simulink model "OneZone_STD2004_Buffalo_TypOcc"  (R2020a)
settings: Solver=FixedStepAuto  StartTime=15638400  StopTime=15811200  FixedStep=60  RelTol=1e-3
settings Model: Creator=zhelu  LastModifiedBy=yl3328

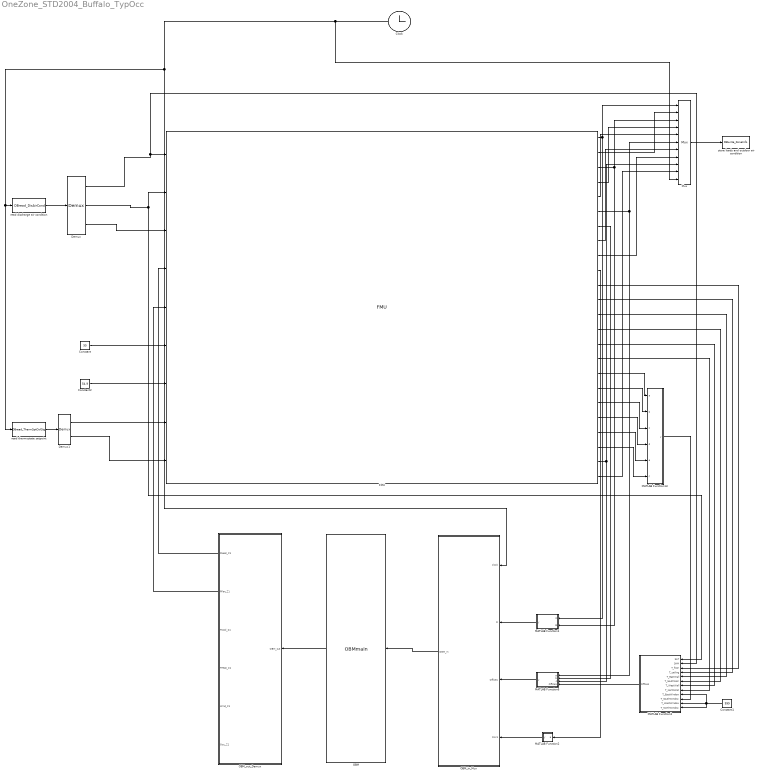
== system OneZone_STD2004_Buffalo_TypOcc ==
  Clock : Clock
  Constant : Constant  Value=55
  Constant1 : Constant  Value=999
  Constant2 : Constant  Value=54.9
  Demux : Demux  Outputs=3
  Demux1 : Demux  Outputs=2
  FMU : FMU  FMUName=ASHRAE901_OfficeSmall_STD2004_Buffalo.fmu  FMUMode=CoSimulation
      mask Type: ASHRAE901_OfficeSmall_STD2004_Buffalo.idf [Co-Simulation, v2.0]
      mask Display:
      | disp('ASHRAE901_OfficeSmall_STD2004_Buffalo.idf');
      | port_label('output',1,'T_out');
      | port_label('output',2,'DewpointT_out');
      | port_label('output',3,'RH_out');
      | port_label('output',4,'Perimeter_ZN_1_SenLoads');
      | port_label('output',5,'Perimeter_ZN_1_LatLoads');
      | port_label('output',6,'Perimeter_ZN_1_Temp');
      | port_label('output',7,'Perimeter_ZN_1_RadTemp');
      | port_label('output',8,'Perimeter_ZN_1_DewpointT');
      | port_label('output',9,'Perimeter_ZN_1_HumdRat');
      | port_label('output',10,'Perimeter_ZN_1_Occ');
      | port_label('output',11,'Perimeter_ZN_1_FLOOR_T');
      | port_label('output',12,'Perimeter_ZN_1_CEILING_T');
      | port_label('output',13,'Perimeter_ZN_1_WALL_EAST_T');
      | port_label('output',14,'Perimeter_ZN_1_WALL_SOUTH_T');
      | port_label('output',15,'Perimeter_ZN_1_WALL_WEST_T');
      | port_label('output',16,'Perimeter_ZN_1_WALL_NORTH_T');
      | port_label('output',17,'Perimeter_ZN_1_WALL_SOUTH_WINDOW1_T');
      | port_label('output',18,'Perimeter_ZN_1_WALL_SOUTH_WINDOW2_T');
      | port_label('output',19,'Perimeter_ZN_1_WALL_SOUTH_WINDOW3_T');
      | port_label('output',20,'Perimeter_ZN_1_WALL_SOUTH_WINDOW4_T');
      | port_label('output',21,'Perimeter_ZN_1_WALL_SOUTH_WINDOW5_T');
      | port_label('output',22,'Perimeter_ZN_1_WALL_SOUTH_WINDOW6_T');
      | port_label('output',23,'Perimeter_ZN_1_RelaHumd');
      | port_label('output',24,'w_out');
      | port_label('input',1,'Perimeter_ZN_1 SupplyFlow');
      | port_label('input',2,'Perimeter_ZN_1 SupplyTemp');
      | port_label('input',3,'Perimeter_ZN_1 SupplyHumd');
      | port_label('input',4,'Perimeter_ZN_1_PHeat');
      | port_label('input',5,'Perimeter_ZN_1_PFan');
      | port_label('input',6,'Perimeter_ZN_1_TCool');
      | port_label('input',7,'Perimeter_ZN_1_THeat');
      | port_label('input',8,'OtherZN_TC');
      | port_label('input',9,'OtherZN_TH');
  MATLAB Function1 : MATLAB Function  TreatAsAtomicUnit=on
  MATLAB Function13 : MATLAB Function  TreatAsAtomicUnit=on
  MATLAB Function2 : MATLAB Function  TreatAsAtomicUnit=on
  MATLAB Function3 : MATLAB Function  TreatAsAtomicUnit=on
  MATLAB Function6 : MATLAB Function  TreatAsAtomicUnit=on
  Mux : Mux  Inputs=11
  OBM : M-S-Function  FunctionName=OBMmain
  OBM_in_Mux : MATLAB Function  TreatAsAtomicUnit=on
  OBM_out_Demux : MATLAB Function  TreatAsAtomicUnit=on
  read discharge air condition : M-S-Function  FunctionName=DBread_DisAirCond
  read thermostate setpoint : M-S-Function  FunctionName=DBread_ThermSptCtrlSig
  store loads and outdoor air condition : M-S-Function  FunctionName=DBwrite_ZoneInfo
  wires:
  Mux/1 -> store loads and outdoor air condition/1
  read discharge air condition/1 -> Demux/1
  Clock/1 -> Mux/11, read thermostate setpoint/1, read discharge air condition/1, OBM_in_Mux/1(clock)
  MATLAB Function1/1(y) -> OBM_in_Mux/2(O)
  MATLAB Function6/1(y) -> OBM_in_Mux/3(Office1)
  MATLAB Function2/1(y) -> OBM_in_Mux/4(Occ1)
  OBM_in_Mux/1(OBM_in) -> OBM/1
  OBM/1 -> OBM_out_Demux/1(OBM_out)
  OBM_out_Demux/1(PHeat_Z1) -> FMU/4
  OBM_out_Demux/2(PFan_Z1) -> FMU/5
  Constant2/1 -> FMU/7
  Constant/1 -> FMU/6
  Demux/1 -> MATLAB Function3/2(SAM), FMU/1
  Demux/2 -> MATLAB Function3/1(SAT), FMU/2
  Demux/3 -> FMU/3
  FMU/1 -> Mux/1, MATLAB Function1/1(A)
  FMU/3 -> MATLAB Function1/2(B), Mux/3
  FMU/10 -> MATLAB Function2/1(a)
  FMU/6 -> MATLAB Function6/1(a), Mux/6
  FMU/7 -> MATLAB Function6/2(b)
  FMU/9 -> Mux/8
  FMU/2 -> Mux/2
  FMU/4 -> Mux/4
  FMU/5 -> Mux/5
  FMU/8 -> Mux/7
  FMU/11 -> MATLAB Function3/3(T_floor)
  FMU/12 -> MATLAB Function3/4(T_ceiling)
  FMU/13 -> MATLAB Function3/5(T_EastWall)
  FMU/14 -> MATLAB Function3/6(T_SouthWall)
  FMU/15 -> MATLAB Function3/7(T_WestWall)
  FMU/16 -> MATLAB Function3/8(T_NorthWall)
  FMU/17 -> MATLAB Function13/1(a)
  FMU/18 -> MATLAB Function13/2(b)
  FMU/19 -> MATLAB Function13/3(c)
  FMU/20 -> MATLAB Function13/4(d)
  FMU/21 -> MATLAB Function13/5(e)
  FMU/22 -> MATLAB Function13/6(f)
  MATLAB Function13/1(y) -> MATLAB Function3/10(T_SouthWindow)
  Constant1/1 -> MATLAB Function3/12(T_NorthWindow), MATLAB Function3/9(T_EastWindow), MATLAB Function3/11(T_WestWindow)
  MATLAB Function3/1(Office1) -> MATLAB Function6/4(Office1)
  FMU/23 -> MATLAB Function6/3(c), Mux/9
  FMU/24 -> Mux/10
  read thermostate setpoint/1 -> Demux1/1
  Demux1/1 -> FMU/8
  Demux1/2 -> FMU/9

== matlab function OneZone_STD2004_Buffalo_TypOcc/MATLAB Function1 ==
  data: A input; y output; B input
function y = fcn(A,B)

y = [A B];

== matlab function OneZone_STD2004_Buffalo_TypOcc/OBM_in_Mux ==
  data: clock input; OBM_in output; O input; Office1 input; Occ1 input
function OBM_in = fcn(clock,O,Office1,Occ1)
% Assemble OBM inputs
OBM_in=[clock,O,Office1,Occ1]';

== matlab function OneZone_STD2004_Buffalo_TypOcc/MATLAB Function2 ==
  data: a input; y output
function y = fcn(a)
if a<0.6
    a=0;
end
a=round(a);
y = [a];

== matlab function OneZone_STD2004_Buffalo_TypOcc/MATLAB Function3 ==
  data: SAT input; SAM input; T_floor input; Office1 output; T_ceiling input; T_EastWall input; T_SouthWall input; T_WestWall input; T_NorthWall input; T_EastWindow input; T_SouthWindow input; T_WestWindow input; T_NorthWindow input
function Office1 = fcn(SAT,SAM,T_floor,T_ceiling,T_EastWall,T_SouthWall,T_WestWall,T_NorthWall,...
    T_EastWindow,T_SouthWindow,T_WestWindow,T_NorthWindow)
Office1=[SAT,SAM,T_floor,T_ceiling,T_EastWall,T_SouthWall,T_WestWall,T_NorthWall,...
    T_EastWindow,T_SouthWindow,T_WestWindow,T_NorthWindow];

== matlab function OneZone_STD2004_Buffalo_TypOcc/MATLAB Function6 ==
  data: a input; y output; b input; c input; Office1 input
function y = fcn(a, b, c, Office1)

y = [a b c Office1];

== matlab function OneZone_STD2004_Buffalo_TypOcc/MATLAB Function13 ==
  data: a input; y output; b input; c input; d input; e input; f input
function y = fcn(a,b,c,d,e,f)
u=(a+b+c+d+e+f)/6;
y = u;

== matlab function OneZone_STD2004_Buffalo_TypOcc/OBM_out_Demux ==
  data: OBM_out input; PHeat_Z1 output; PFan_Z1 output; TCool_Z1 output; THeat_Z1 output; Wind_Z1 output; Occ_Z1 output
function [PHeat_Z1,PFan_Z1,TCool_Z1,THeat_Z1,Wind_Z1,Occ_Z1] = fcn(OBM_out)

PHeat_Z1 = OBM_out(1);
PFan_Z1 = OBM_out(2);
TCool_Z1 = OBM_out(3);
THeat_Z1 = OBM_out(4);
Wind_Z1 = OBM_out(5);
Occ_Z1 = OBM_out(6);
